simulink model "cortical_basal_ganglia_circuit"  (R2021a)
settings: Solver=VariableStepAuto  StartTime=0.0  StopTime=5  RelTol=1e-3
values from neighbouring files (symbols this model uses):
  D2_GPe = 0.5*C_bg_th    (= 30)    [circuit_parameters.m]
  EI_PY = 4.8*C_cor    (= 288)    [circuit_parameters.m]
  GPe_GPe = 0.5*C_bg_th    (= 30)    [circuit_parameters.m]
  GPe_GPi = 0.5*C_bg_th    (= 30)    [circuit_parameters.m]
  GPe_STN = 0.5*C_bg_th    (= 30)    [circuit_parameters.m]
  GPi_Th = 0.5*C_bg_th    (= 30)    [circuit_parameters.m]
  H_d2 = 20    [circuit_parameters.m]
  H_EI = 20    [circuit_parameters.m]
  H_g = 20    [circuit_parameters.m]
  H_gi = 20    [circuit_parameters.m]
  H_II = 60    [circuit_parameters.m]
  H_PY = 20    [circuit_parameters.m]
  H_s = 20    [circuit_parameters.m]
  H_t = 10    [circuit_parameters.m]
  II_II = 3.3*C_cor    (= 198)    [circuit_parameters.m]
  II_PY = 1.5*C_cor    (= 90)    [circuit_parameters.m]
  PY_EI = 6*C_cor    (= 360)    [circuit_parameters.m]
  PY_II = 1.5*C_cor    (= 90)    [circuit_parameters.m]
  PY_STN = C_cor_bg_th    (= 5)    [circuit_parameters.m]
  STN_GPe = C_bg_th    (= 60)    [circuit_parameters.m]
  tau_d2 = 0.0022    [circuit_parameters.m]
  tau_EI = 0.01    [circuit_parameters.m]
  tau_g = 0.014    [circuit_parameters.m]
  tau_gi = 0.014    [circuit_parameters.m]
  tau_II = 2    [circuit_parameters.m]
  tau_PY = 0.001    [circuit_parameters.m]
  tau_s = 0.01    [circuit_parameters.m]
  tau_t = 0.002    [circuit_parameters.m]
  Th_EI = C_bg_th_cor    (= 5)    [circuit_parameters.m]
settings Model: Creator=Vitoria Fahed  LastModifiedBy=senne
settings SolverCC: AlgebraicLoopSolver=TrustRegion
settings DebuggingCC: SFMachineParentedDataDiag=warning

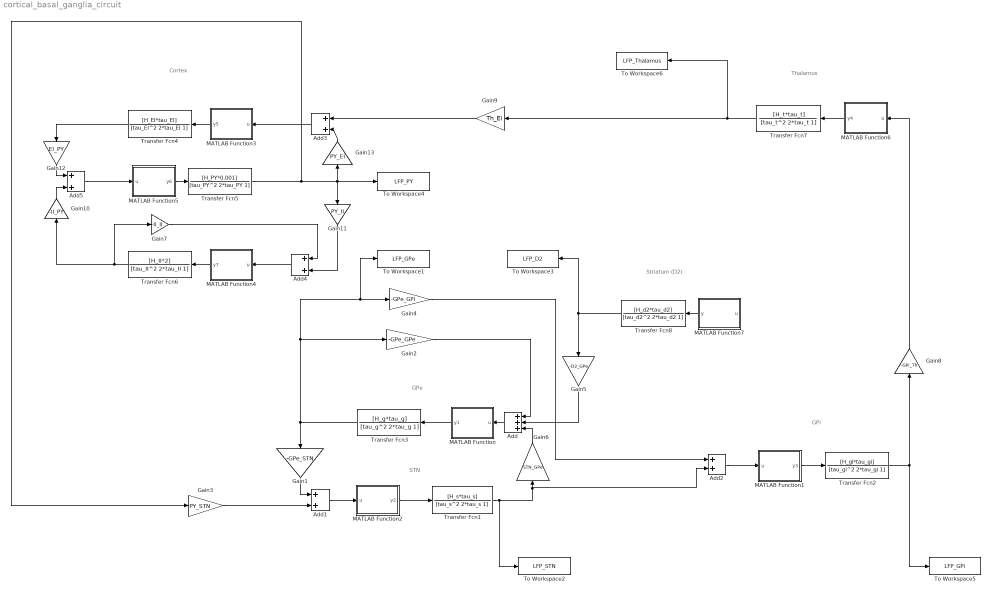
== system cortical_basal_ganglia_circuit ==
  note: GPe
  note: STN
  note: Striatum (D2)
  note: Cortex
  note: GPi
  note: Thalamus
  Add : Sum  Inputs=+++
  Add{1..5} (5 alike) : Sum
  Gain1 : Gain  Gain=-GPe_STN
  Gain10 : Gain  Gain=-II_PY
  Gain11 : Gain  Gain=PY_II
  Gain12 : Gain  Gain=EI_PY
  Gain13 : Gain  Gain=PY_EI
  Gain2 : Gain  Gain=-GPe_GPe
  Gain3 : Gain  Gain=PY_STN
  Gain4 : Gain  Gain=-GPe_GPi
  Gain5 : Gain  Gain=-D2_GPe
  Gain6 : Gain  Gain=STN_GPe
  Gain7 : Gain  Gain=-II_II
  Gain8 : Gain  Gain=-GPi_Th
  Gain9 : Gain  Gain=Th_EI
  MATLAB Function : MATLAB Function  TreatAsAtomicUnit=on
  MATLAB Function1 : MATLAB Function  TreatAsAtomicUnit=on
  MATLAB Function2 : MATLAB Function  TreatAsAtomicUnit=on
  MATLAB Function3 : MATLAB Function  TreatAsAtomicUnit=on
  MATLAB Function4 : MATLAB Function  TreatAsAtomicUnit=on
  MATLAB Function5 : MATLAB Function  TreatAsAtomicUnit=on
  MATLAB Function6 : MATLAB Function  TreatAsAtomicUnit=on
  MATLAB Function7 : MATLAB Function  TreatAsAtomicUnit=on
  To Workspace1 : ToWorkspace  VariableName=LFP_GPe  SaveFormat=Timeseries  SampleTime=-1
  To Workspace2 : ToWorkspace  VariableName=LFP_STN  SaveFormat=Timeseries  SampleTime=-1
  To Workspace3 : ToWorkspace  VariableName=LFP_D2  SaveFormat=Timeseries  SampleTime=-1
  To Workspace4 : ToWorkspace  VariableName=LFP_PY  SaveFormat=Timeseries  SampleTime=-1
  To Workspace5 : ToWorkspace  VariableName=LFP_GPi  SaveFormat=Timeseries  SampleTime=-1
  To Workspace6 : ToWorkspace  VariableName=LFP_Thalamus  SaveFormat=Timeseries  SampleTime=-1
  Transfer Fcn1 : TransferFcn  Numerator=[H_s*tau_s]  Denominator=[tau_s^2 2*tau_s 1]
  Transfer Fcn2 : TransferFcn  Numerator=[H_gi*tau_gi]  Denominator=[tau_gi^2 2*tau_gi 1]
  Transfer Fcn3 : TransferFcn  Numerator=[H_g*tau_g]  Denominator=[tau_g^2 2*tau_g 1]
  Transfer Fcn4 : TransferFcn  Numerator=[H_EI*tau_EI]  Denominator=[tau_EI^2 2*tau_EI 1]
  Transfer Fcn5 : TransferFcn  Numerator=[H_PY*0.001]  Denominator=[tau_PY^2 2*tau_PY 1]
  Transfer Fcn6 : TransferFcn  Numerator=[H_II*2]  Denominator=[tau_II^2 2*tau_II 1]
  Transfer Fcn7 : TransferFcn  Numerator=[H_t*tau_t]  Denominator=[tau_t^2 2*tau_t 1]
  Transfer Fcn8 : TransferFcn  Numerator=[H_d2*tau_d2]  Denominator=[tau_d2^2 2*tau_d2 1]
  wires:
  MATLAB Function2/1(y2) -> Transfer Fcn1/1
  Transfer Fcn1/1 -> To Workspace2/1, Add2/2, Gain6/1
  Add/1 -> MATLAB Function/1(u)
  Transfer Fcn3/1 -> To Workspace1/1, Gain4/1, Gain2/1, Gain1/1
  Gain5/1 -> Add/2
  MATLAB Function/1(y1) -> Transfer Fcn3/1
  Gain6/1 -> Add/3
  Gain2/1 -> Add/1
  Gain1/1 -> Add1/1
  Add1/1 -> MATLAB Function2/1(u)
  Gain3/1 -> Add1/2
  MATLAB Function1/1(y3) -> Transfer Fcn2/1
  Gain4/1 -> Add2/1
  Add2/1 -> MATLAB Function1/1(u)
  MATLAB Function3/1(y5) -> Transfer Fcn4/1
  MATLAB Function5/1(y6) -> Transfer Fcn5/1
  MATLAB Function4/1(y7) -> Transfer Fcn6/1
  Transfer Fcn6/1 -> Gain10/1, Gain7/1
  MATLAB Function6/1(y4) -> Transfer Fcn7/1
  MATLAB Function7/1(y) -> Transfer Fcn8/1
  Transfer Fcn8/1 -> Gain5/1, To Workspace3/1
  Transfer Fcn7/1 -> To Workspace6/1, Gain9/1
  Transfer Fcn2/1 -> To Workspace5/1, Gain8/1
  Gain8/1 -> MATLAB Function6/1(u)
  Gain9/1 -> Add3/1
  Transfer Fcn5/1 -> To Workspace4/1, Gain13/1, Gain11/1, Gain3/1
  Add3/1 -> MATLAB Function3/1(u)
  Gain7/1 -> Add4/1
  Add4/1 -> MATLAB Function4/1(u)
  Transfer Fcn4/1 -> Gain12/1
  Gain10/1 -> Add5/2
  Add5/1 -> MATLAB Function5/1(u)
  Gain11/1 -> Add4/2
  Gain12/1 -> Add5/1
  Gain13/1 -> Add3/2

== matlab function cortical_basal_ganglia_circuit/MATLAB Function ==
  data: u input; y1 output
function y1 = GPe_NL(u)
gamma_g = 400;
r_g = 0.1;
y1 = gamma_g/(1 + exp(-r_g*u));

== matlab function cortical_basal_ganglia_circuit/MATLAB Function2 ==
  data: u input; y2 output
function y2 = STN_NL(u)
gamma_s = 500;
r_s = 0.1;
y2 = gamma_s/(1 + exp(-r_s*u));

== matlab function cortical_basal_ganglia_circuit/MATLAB Function3 ==
  data: u input; y5 output
function y5 = EI_NL(u)
gamma_EI = 5;
r_EI = 5;
y5 = gamma_EI/(1 + exp(-r_EI*u));

== matlab function cortical_basal_ganglia_circuit/MATLAB Function4 ==
  data: u input; y7 output
function y7 = II_NL(u)
gamma_II = 5;
r_II = 5;
y7 = gamma_II/(1 + exp(-r_II*u));

== matlab function cortical_basal_ganglia_circuit/MATLAB Function5 ==
  data: u input; y6 output
function y6 = PY_NL(u)
gamma_PY = 5;
r_PY = 0.15;
y6 = gamma_PY/(1 + exp(-r_PY*u));

== matlab function cortical_basal_ganglia_circuit/MATLAB Function6 ==
  data: u input; y4 output
function y4 = Th_NL(u)
gamma_t = 20;
r_t = 5;
y4 = gamma_t/(1 + exp(-r_t*u));

== matlab function cortical_basal_ganglia_circuit/MATLAB Function7 ==
  data: u input; y output
function y = D2_NL(u)
gamma_d2 = 300;
r_d2 = 0.3;
y = gamma_d2/(1 + exp(-r_d2*u));

== matlab function cortical_basal_ganglia_circuit/MATLAB Function1 ==
  data: u input; y3 output
function y3 = GPi_NL(u)
gamma_gi = 400;
r_gi = 0.1;
y3 = gamma_gi/(1 + exp(-r_gi*u));
